simulink model "lab1_model"  (Simulink 7.6)
settings: Solver=ode45  StartTime=0.0  StopTime=1500  RelTol=1e-3
values from neighbouring files (symbols this model uses):
  cpw = 4190    [Spawek_ch_dyn.m]    (also in lab1_chki_dyn.m; lab1_skrypt.m; lab2_skrypt.m)
  Cvg = cpw*row*Vg/4    (= 20531)    [Spawek_ch_dyn.m]    (also in lab1_chki_dyn.m; lab1_skrypt.m)
  Cvw = cpp*rop*Vp    (= 23889.6)    [Spawek_ch_dyn.m]    (also in lab1_chki_dyn.m; lab1_skrypt.m)
  dFg = dFg_    [Spawek_ch_dyn.m]    (also in Spawek_script.m = 0.0001; lab1_chki_dyn.m = 0; lab1_skrypt.m = 0; lab2_skrypt.m = 0)
  dQt = dQt_    [Spawek_ch_dyn.m]    (also in Spawek_script.m = 0; lab1_chki_dyn.m = 0; lab1_skrypt.m = 0; lab2_skrypt.m = 0)
  dt = 0    [Spawek_ch_dyn.m]    (also in lab1_chki_dyn.m; lab1_skrypt.m = 100; lab2_skrypt.m = 5)
  dTgz = dTgz_    [Spawek_ch_dyn.m]    (also in Spawek_script.m = 0; lab1_chki_dyn.m = 0; lab1_skrypt.m = 0; lab2_skrypt.m = 0)
  dTzew = dTzew_    [Spawek_ch_dyn.m]    (also in Spawek_script.m = 0; lab1_chki_dyn.m = 10; lab1_skrypt.m = 0; lab2_skrypt.m = 0)
  Fg_0 = Fg_n    [Spawek_ch_dyn.m]    (also in lab1_chki_dyn.m = 0.000243534167844; lab1_skrypt.m = 0.000243534167844; lab2_skrypt.m = 0.000243534167844)
  kg = Q_n/(Tgsr_n-Twew_n) * fg_mod    [Spawek_ch_dyn.m]    (also in lab1_chki_dyn.m = 400; lab1_skrypt.m = 400; lab2_skrypt.m = 400)
  kw = (Q_n-Qt_n)/(Twew_n-Tzew_n) * fg_mod    [Spawek_ch_dyn.m]    (also in lab1_chki_dyn.m = 500; lab1_skrypt.m = 500; lab2_skrypt.m = 500)
  Qt_0 = Qt_n    (= 0)    [Spawek_ch_dyn.m]    (also in lab1_chki_dyn.m; lab1_skrypt.m; lab2_skrypt.m)
  row = 980    [Spawek_ch_dyn.m]    (also in lab1_chki_dyn.m; lab1_skrypt.m; lab2_skrypt.m)
  Tgsr_0 = Tgsr_n    (= 70)    [Spawek_ch_dyn.m]    (also in lab1_chki_dyn.m; lab1_skrypt.m; lab2_skrypt.m)
  Tgz_0 = Tgz_n    [Spawek_ch_dyn.m]    (also in lab1_chki_dyn.m = 90; lab1_skrypt.m = 90; lab2_skrypt.m = 90)
  Twew_0 = Twew_n    (= 20)    [Spawek_ch_dyn.m]    (also in lab1_chki_dyn.m; lab1_skrypt.m; lab2_skrypt.m)
  Tzew_0 = Tzew_n    [Spawek_ch_dyn.m]    (also in lab1_chki_dyn.m = -20; lab1_skrypt.m = -20; lab2_skrypt.m = -18)
settings Model: Creator=LAB320-1537-User  LastModifiedBy=qrczak
settings DebuggingCC: FcnCallInpInsideContextMsg=Enable All
settings GRTTargetCC: CombineOutputUpdateFcns=on

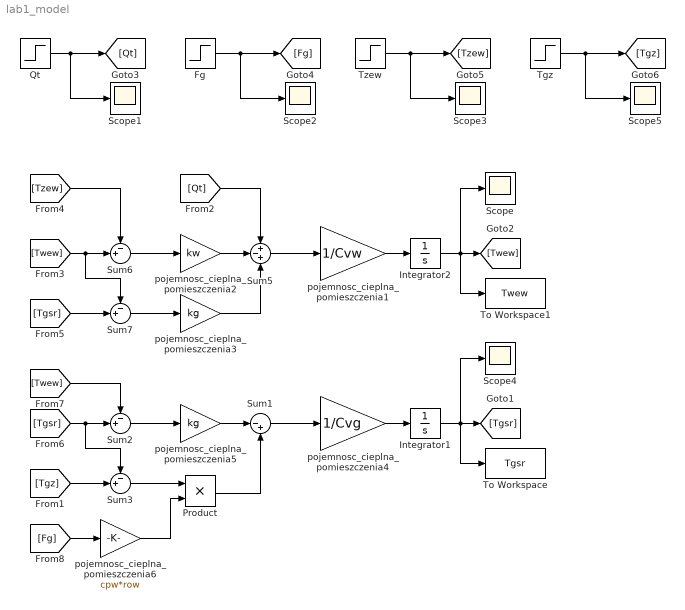
== system lab1_model ==
  Fg : Step  Time=dt  Before=Fg_0  After=Fg_0+dFg  SampleTime=0
  Integrator1 : Integrator  InitialCondition=Tgsr_0
  Integrator2 : Integrator  InitialCondition=Twew_0
  Product : Product  RndMeth=Zero
  Qt : Step  Time=dt  Before=Qt_0  After=Qt_0+dQt  SampleTime=0
  Scope{,1..5} (6 alike) : Scope
      Scope settings: SaveName=ScopeData2
      Scope1 settings: SaveName=ScopeData3
      Scope3 settings: SaveName=ScopeData5
      Scope5 settings: SaveName=ScopeData4
  Sum1 : Sum  Inputs=|-+
  Sum{2..3,6..7} (4 alike) : Sum  Inputs=-+|
  Sum5 : Sum  Inputs=+-+
  Tgz : Step  Time=dt  Before=Tgz_0  After=Tgz_0+dTgz  SampleTime=0
  To Workspace : ToWorkspace  VariableName=Tgsr  SampleTime=-1  SaveFormat=Structure With Time
  To Workspace1 : ToWorkspace  VariableName=Twew  SampleTime=-1  SaveFormat=Structure With Time
  Tzew : Step  Time=dt  Before=Tzew_0  After=Tzew_0+dTzew  SampleTime=0
  pojemnosc_cieplna_pomieszczenia1 : Gain  Gain=1/Cvw
  pojemnosc_cieplna_pomieszczenia2 : Gain  Gain=kw
  pojemnosc_cieplna_pomieszczenia3 : Gain  Gain=kg
  pojemnosc_cieplna_pomieszczenia4 : Gain  Gain=1/Cvg
  pojemnosc_cieplna_pomieszczenia5 : Gain  Gain=kg
  pojemnosc_cieplna_pomieszczenia6 : Gain  Gain=cpw*row
  wires:
  pojemnosc_cieplna_pomieszczenia1/1 -> Integrator2/1
  Integrator2/1 -> [Twew], Scope/1, To Workspace1/1
  Qt/1 -> [Qt], Scope1/1
  Tzew/1 -> Scope3/1, [Tzew]
  Sum5/1 -> pojemnosc_cieplna_pomieszczenia1/1
  [Qt] -> Sum5/1
  pojemnosc_cieplna_pomieszczenia2/1 -> Sum5/2
  pojemnosc_cieplna_pomieszczenia3/1 -> Sum5/3
  Sum6/1 -> pojemnosc_cieplna_pomieszczenia2/1
  [Twew] -> Sum6/2, Sum7/1
  [Tzew] -> Sum6/1
  [Tgsr] -> Sum7/2
  Sum7/1 -> pojemnosc_cieplna_pomieszczenia3/1
  pojemnosc_cieplna_pomieszczenia4/1 -> Integrator1/1
  Integrator1/1 -> [Tgsr], Scope4/1, To Workspace/1
  Sum1/1 -> pojemnosc_cieplna_pomieszczenia4/1
  Sum2/1 -> pojemnosc_cieplna_pomieszczenia5/1
  [Tgsr] -> Sum2/2, Sum3/1
  [Twew] -> Sum2/1
  pojemnosc_cieplna_pomieszczenia5/1 -> Sum1/1
  [Tgz] -> Sum3/2
  [Fg] -> pojemnosc_cieplna_pomieszczenia6/1
  pojemnosc_cieplna_pomieszczenia6/1 -> Product/2
  Sum3/1 -> Product/1
  Product/1 -> Sum1/2
  Fg/1 -> Scope2/1, [Fg]
  Tgz/1 -> Scope5/1, [Tgz]
